simulink model "Part2_Updated_2024a"  (R2024a)
settings: Solver=FixedStepAuto  StartTime=0.0  StopTime=300  FixedStep=0.1  RelTol=1e-3
values from neighbouring files (symbols this model uses):
  Af = [0.1,0.1,0.01]    [init_Updated.m]
  Aw = [zeros(3,3), eye(3); diag(-0.3948*[1 1 1]), diag(-0.0126*[1 1 1])]    [init_Updated.m]
  B = [0,1,0,0,1,0,1,0 ... (first row only)    [init_Updated.m]
  Cw = [zeros(3) eye(3)]    [init_Updated.m]
  D = [2.6486e5, 0, 0 ... (first row only)    [init_Updated.m]
  eta0 = [0,0,0,0,0,0]'    [init_Updated.m]
  Gamma = [omega(1)^2,omega(2)^2,omega(3)^2]    [init_Updated.m]
  K1 = [diag(-3.762*[1 1 1]); diag(1.2441*[1 1 1])]    [init_Updated.m]
  K2 = diag(1.1938*[1 1 1])    [init_Updated.m]
  K3 = diag([3.57e5 3.57e5 3.57e7])    [init_Updated.m]
  K4 = 10*K3    [init_Updated.m]
  Kd = -[-885551.128894883; -1413618.40984523; -582749740.806195]    [init_Updated.m]
  Ki = -[-540.64009360768; -3153.2361136748; -1036593.12054623]    [init_Updated.m]
  Kp = -[-44440.8471205421; -174748.115243117; -56099945.0910478]    [init_Updated.m]
  M = [7.0101e6, 0, 0 ... (first row only)    [init_Updated.m]
  mu_current = 0.0001    [init_Updated.m]
  mu_current_dir = 0.001    [init_Updated.m]
  mu_dir = 0    [init_Updated.m]
  mu_speed = 0.001    [init_Updated.m]
  n = 21    [init_Updated.m]
  nu_c = 0.2    [init_Updated.m]
  omega = [2*zeta*2*pi/10,2*zeta*2*pi/10,2*zeta*2*pi/10]    [init_Updated.m]
  psi_c = n*10*pi/180    (= 3.66519142919)    [init_Updated.m]
  simulation = 2    [init_Updated.m]
  T = diag(10e3*[1 1 1])    [init_Updated.m]
  U_10 = 12    [init_Updated.m]
  U_mean = U_10 * (5 / 2 )* sqrt(kappa) * log(z / z0)    [init_Updated.m]
  Umean_angle = n*10    (= 210)    [init_Updated.m]
undefined symbols (not defined in the file or in its folder): Hoerner, thrusters, vessel, wind_coeff
libraries: simulink x11, simulink_extras x3, dspsigops x3, marine_hydro x2, marine_gnc x1
settings Model: Creator=jonbjor  LastModifiedBy=HP
settings SolverCC: AlgebraicLoopSolver=TrustRegion
settings DataIOCC: ReturnWorkspaceOutputs=off
settings DebuggingCC: UnconnectedInputMsg=warning  UnconnectedOutputMsg=warning  UnconnectedLineMsg=warning  ArithmeticOperatorsInVariantConditions=warning
settings ModelReferenceCC: EnableRefExpFcnMdlSchedulingChecks=on
settings SFSimCC: SimUseLocalCustomCode=off  CustomCodeUndefinedFunction=UseInterfaceOnly
settings RTWCC: RTWUseLocalCustomCode=off  GPUComputeCapability=3.5  DLArmComputeVersion=19.05

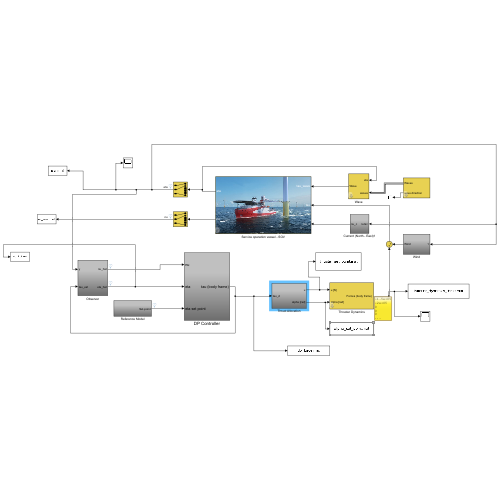
[thumbnail: Simulink's stored preview of the top-level diagram]
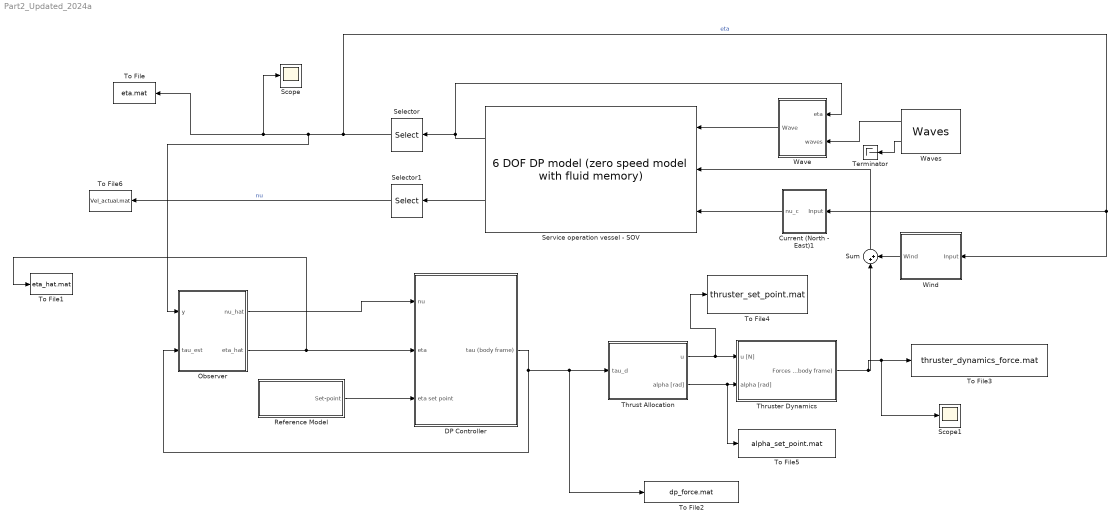
== system Part2_Updated_2024a ==
  Current (North - East)1 : Subsystem
  DP Controller : Subsystem
  Observer : Subsystem
  Reference Model : Subsystem
  Scope : Scope
  Scope1 : Scope
  Selector : Selector  InputPortWidth=6  IndexOptions=Index vector (dialog)  Indices=[1 2 6]  OutputSizes=1
  Selector1 : Selector  InputPortWidth=6  IndexOptions=Index vector (dialog)  Indices=[1 2 6]  OutputSizes=1
  Service operation vessel - SOV : marine_hydro/Hydro Library/6 DOF DP model  (zero speed model with fluid memory)  ABC=vesselABC  rho=1025  Axc=0.9*vessel.main.T*vessel.main.B  Ayc=0.9*vessel.main.T*vessel.main.Lpp  CX=1  CY_2D=Hoerner(vessel.main.B,vessel.main.T)  Bv=vessel.Bv  mask(6 DOF zero speed model){}
      mask Display:
      | image('SOV.jpg');
      | color('white'); port_label('output', 1, 'eta')
      | color('white'); port_label('output', 2, 'nu')
      | color('white'); port_label('input', 1, 'tau_wave')
      | color('white'); port_label('input', 2, 'tau')
      | color('white'); port_label('input', 3, 'nu_c')
  Sum : Sum  Inputs=|++
  Terminator : Terminator
  Thrust Allocation : Subsystem
  Thruster Dynamics : Subsystem  mask{thrusterfault=off}
      mask prompts: thrusterfault "Fault on thruster #2 and #4?"
  To File : ToFile  Filename=eta.mat  MatrixName=Track  SaveFormat=Timeseries
  To File1 : ToFile  Filename=eta_hat.mat  MatrixName=eta_hat  SaveFormat=Timeseries
  To File2 : ToFile  Filename=dp_force.mat  MatrixName=dp  SaveFormat=Timeseries
  To File3 : ToFile  Filename=thruster_dynamics_force.mat  MatrixName=thruter  SaveFormat=Timeseries
  To File4 : ToFile  Filename=thruster_set_point.mat  MatrixName=thrusterset  SaveFormat=Timeseries
  To File5 : ToFile  Filename=alpha_set_point.mat  MatrixName=alpha  SaveFormat=Timeseries
  To File6 : ToFile  Filename=Vel_actual.mat  MatrixName=Vel_actual  SaveFormat=Timeseries
  Wave : Subsystem  mask{waveforces=on}
      mask prompts: waveforces "Waveforces enabled"
  Waves : marine_gnc/Environment/Waves/Waves  spectrum_type=ITTC  disp_flag=on  plot_spectrum=off  plot_realization=off  hs=4  omega_peak=2*pi/3  psi_mean=n*10*pi/180  gamma=-1  spread=2  depth=inf  nfreq=20  ndir=10  energylim=0.005  freq_cutoff=3  dir_cutoff=0  rand_seed=123  rand_freq=on  rand_dir=on  Zeta_a=0  Omega=0  Phase=0  Wavenum=0  Psi=0
  Wind : Subsystem
  wires:
  Service operation vessel - SOV/1 -> Wave/1(eta), Selector/1
  Service operation vessel - SOV/2 -> Selector1/1
  Selector/1 -> Observer/1(y), Scope/1, To File/1, Wind/1(Input), Current (North - East)1/1(Input)  "eta"
  Thrust Allocation/1(u) -> To File4/1, Thruster Dynamics/1(u [N])
  Thrust Allocation/2(alpha [rad]) -> To File5/1, Thruster Dynamics/2(alpha [rad])
  Sum/1 -> Service operation vessel - SOV/2
  Reference Model/1(Set-point) -> DP Controller/3(eta set point)
  Waves/1 -> Wave/2(waves)
  Waves/2 -> Terminator/1
  Thruster Dynamics/1("Forces (body frame) ") -> Sum/1, Scope1/1, To File3/1
  Selector1/1 -> To File6/1  "nu"
  Observer/2(eta_hat) -> DP Controller/2(eta), To File1/1
  DP Controller/1(tau (body frame)) -> Observer/2(tau_est), To File2/1, Thrust Allocation/1(tau_d)
  Wave/1(Wave) -> Service operation vessel - SOV/1
  Current (North - East)1/1(nu_c) -> Service operation vessel - SOV/3
  Wind/1(Wind) -> Sum/2
  Observer/1(nu_hat) -> DP Controller/1(nu)

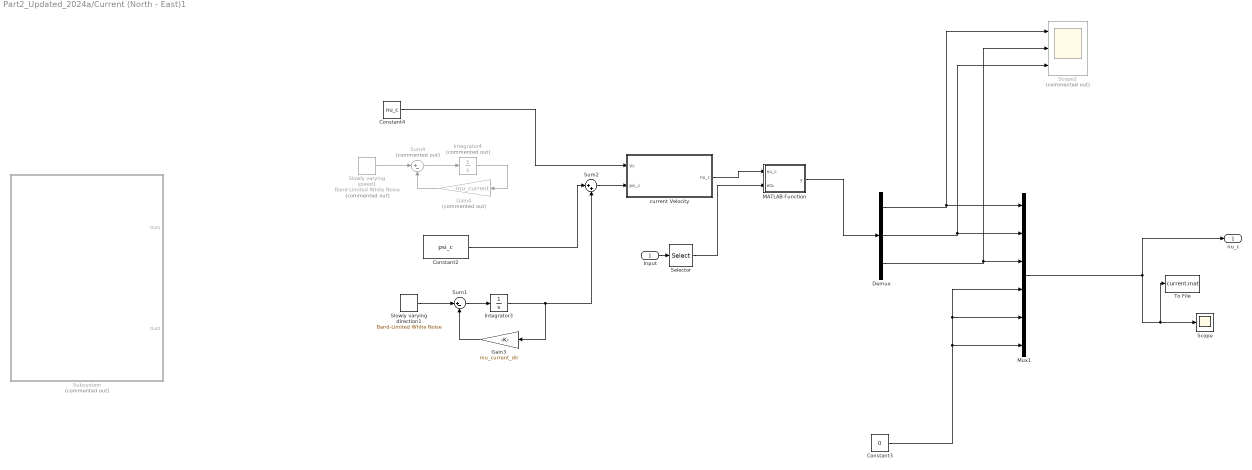
== system Part2_Updated_2024a/Current (North - East)1 ==
  Input : Inport
  Constant2 : Constant  Value=psi_c
  Constant3 : Constant  Value=0
  Constant4 : Constant  Value=nu_c
  Demux : Demux  Outputs=3
  Gain3 : Gain  Gain=mu_current_dir
  Gain4 : Gain  Commented=on  Gain=mu_current
  Integrator3 : Integrator
  Integrator4 : Integrator  Commented=on
  MATLAB Function : MATLAB Function  TreatAsAtomicUnit=on
  Mux1 : Mux  Inputs=6
  Scope : Scope
  Scope2 : Scope  Commented=on  NumInputPorts=3
  Selector : Selector  InputPortWidth=3  IndexOptions=Index vector (dialog)  Indices=[3]  OutputSizes=1
  Slowly varying speed1 : simulink/Sources/Band-Limited White Noise  Commented=on  Cov=[0.001]  Ts=0.1  seed=[23341]
  Slowly varying direction1 : simulink/Sources/Band-Limited White Noise  Cov=[0.0000001]  Ts=0.1  seed=[23341]
  Subsystem : Subsystem  Commented=on
  Sum1 : Sum  Inputs=|+-
  Sum2 : Sum  Inputs=|++
  Sum4 : Sum  Commented=on  Inputs=|+-
  To File : ToFile  Filename=current.mat  MatrixName=current  SaveFormat=Timeseries
  current Velocity : MATLAB Function  TreatAsAtomicUnit=on
  nu_c : Outport
  wires:
  Demux/1 -> Mux1/1, Scope2/1
  Demux/2 -> Mux1/2, Scope2/3
  Demux/3 -> Mux1/3, Scope2/2
  Constant3/1 -> Mux1/4, Mux1/5, Mux1/6
  current Velocity/1(nu_c) -> MATLAB Function/1(nu_c)
  Mux1/1 -> To File/1, Scope/1, nu_c/1
  MATLAB Function/1(y) -> Demux/1
  Input/1 -> Selector/1
  Sum1/1 -> Integrator3/1
  Slowly varying direction1/1 -> Sum1/1
  Integrator3/1 -> Sum2/2, Gain3/1
  Gain3/1 -> Sum1/2
  Constant2/1 -> Sum2/1
  Sum2/1 -> current Velocity/2(psi_c)
  Sum4/1 -> Integrator4/1
  Slowly varying speed1/1 -> Sum4/1
  Integrator4/1 -> Gain4/1
  Gain4/1 -> Sum4/2
  Constant4/1 -> current Velocity/1(Vc)
  Selector/1 -> MATLAB Function/2(eta)

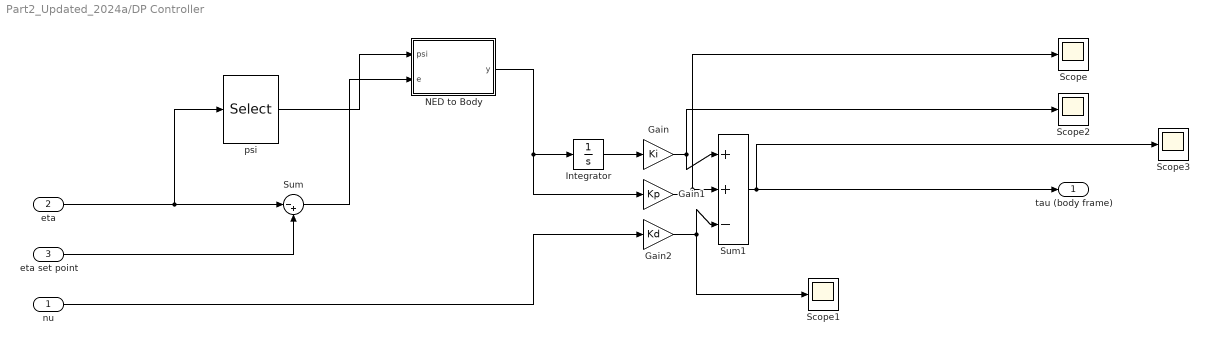
== system Part2_Updated_2024a/DP Controller ==
  nu : Inport
  eta : Inport  Port=2
  eta set point : Inport  Port=3
  Gain : Gain  Gain=Ki
  Gain1 : Gain  Gain=Kp
  Gain2 : Gain  Gain=Kd
  Integrator : Integrator
  "NED to Body " : MATLAB Function  TreatAsAtomicUnit=on
  Scope{,1..3} (4 alike) : Scope
  Sum : Sum  Inputs=|-+
  Sum1 : Sum  Inputs=|++-|
  psi : Selector  InputPortWidth=3  IndexOptions=Index vector (dialog)  Indices=[3]  OutputSizes=1
  tau (body frame) : Outport  VectorParamsAs1DForOutWhenUnconnected=off
  wires:
  Integrator/1 -> Gain/1
  eta/1 -> Sum/1, psi/1
  Sum1/1 -> tau (body frame)/1, Scope3/1
  nu/1 -> Gain2/1
  Gain/1 -> Scope2/1, Sum1/1
  Gain2/1 -> Scope1/1, Sum1/3
  Gain1/1 -> Scope/1, Sum1/2
  Sum/1 -> "NED to Body "/2(e)
  psi/1 -> "NED to Body "/1(psi)
  eta set point/1 -> Sum/2
  "NED to Body "/1(y) -> Gain1/1, Integrator/1

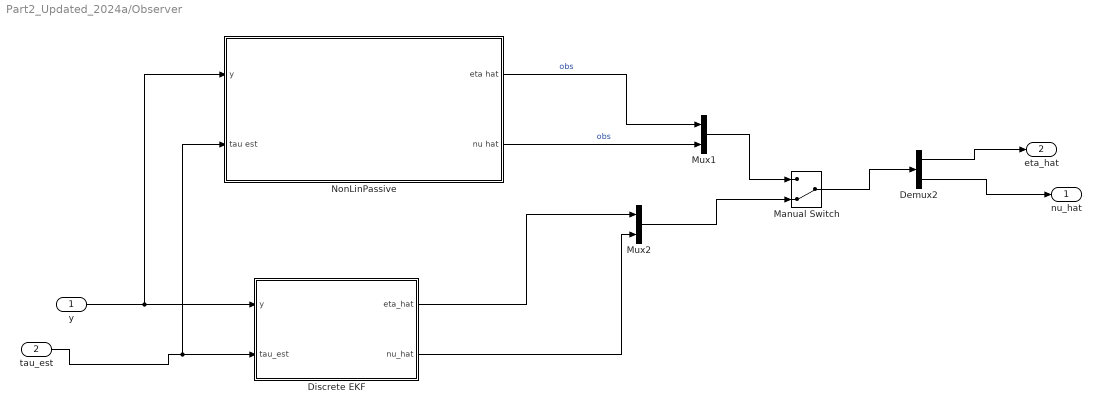
== system Part2_Updated_2024a/Observer ==
  y : Inport
  tau_est : Inport  Port=2
  Demux2 : Demux  Outputs=2
  Discrete EKF : Subsystem
  Manual Switch : ManualSwitch  CurrentSetting=0
  Mux1 : Mux  Inputs=2
  Mux2 : Mux  Inputs=2
  NonLinPassive : Subsystem
  nu_hat : Outport  VectorParamsAs1DForOutWhenUnconnected=off
  eta_hat : Outport  Port=2  VectorParamsAs1DForOutWhenUnconnected=off
  wires:
  y/1 -> Discrete EKF/1(y), NonLinPassive/1(y)
  Mux1/1 -> Manual Switch/1
  Mux2/1 -> Manual Switch/2
  Manual Switch/1 -> Demux2/1
  Demux2/1 -> eta_hat/1
  Demux2/2 -> nu_hat/1
  tau_est/1 -> Discrete EKF/2(tau_est), NonLinPassive/2(tau est)
  Discrete EKF/1(eta_hat) -> Mux2/1
  Discrete EKF/2(nu_hat) -> Mux2/2
  NonLinPassive/1(eta hat) -> Mux1/1  "obs"
  NonLinPassive/2(nu hat) -> Mux1/2  "obs"

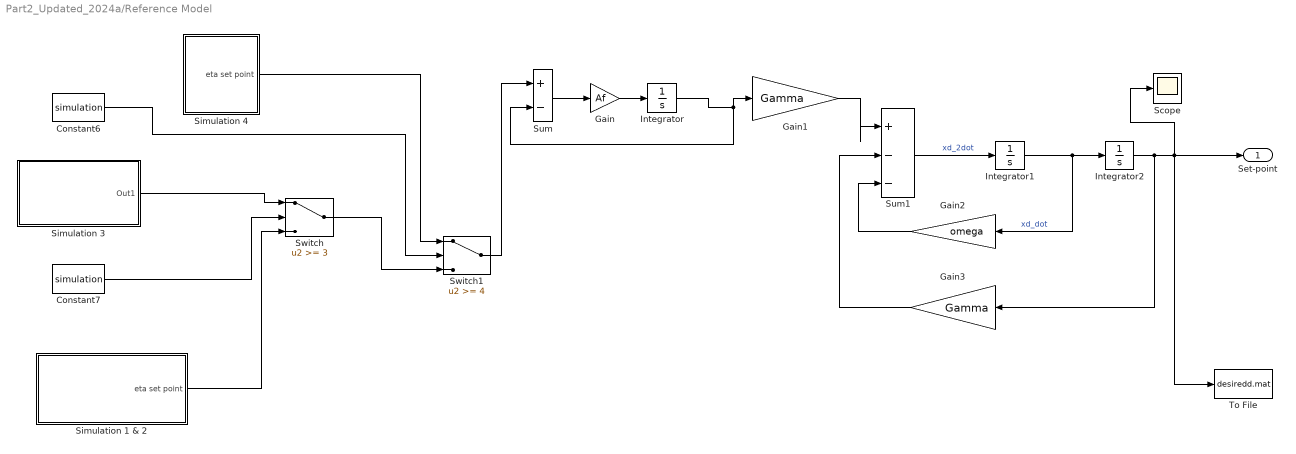
== system Part2_Updated_2024a/Reference Model ==
  Constant6 : Constant  Value=simulation
  Constant7 : Constant  Value=simulation
  Gain : Gain  Gain=Af
  Gain1 : Gain  Gain=Gamma
  Gain2 : Gain  Gain=omega
  Gain3 : Gain  Gain=Gamma
  Integrator : Integrator
  Integrator1 : Integrator
  Integrator2 : Integrator
  Scope : Scope
  Simulation 1 & 2 : Subsystem
  Simulation 3 : Subsystem
  Simulation 4 : Subsystem
  Sum : Sum  Inputs=+-
  Sum1 : Sum  Inputs=|+--
  Switch : Switch  Threshold=3  SaturateOnIntegerOverflow=off  InputSameDT=off
  Switch1 : Switch  Threshold=4  SaturateOnIntegerOverflow=off  InputSameDT=off
  To File : ToFile  Filename=desiredd.mat  MatrixName=Reff  SaveFormat=Timeseries
  Set-point : Outport  VectorParamsAs1DForOutWhenUnconnected=off
  wires:
  Gain/1 -> Integrator/1
  Sum/1 -> Gain/1
  Integrator/1 -> Sum/2, Gain1/1
  Sum1/1 -> Integrator1/1  "xd_2dot"
  Integrator1/1 -> Integrator2/1, Gain2/1  "xd_dot"
  Integrator2/1 -> Scope/1, To File/1, Set-point/1, Gain3/1
  Gain2/1 -> Sum1/3
  Gain3/1 -> Sum1/2
  Gain1/1 -> Sum1/1
  Switch1/1 -> Sum/1
  Simulation 4/1(eta set point) -> Switch1/1
  Switch/1 -> Switch1/3
  Simulation 3/1(Out1) -> Switch/1
  Constant7/1 -> Switch/2
  Constant6/1 -> Switch1/2
  Simulation 1 & 2/1(eta set point) -> Switch/3

== system Part2_Updated_2024a/Thrust Allocation ==
  tau_d : Inport
  Constant : Constant  Value=B
  MATLAB Function : MATLAB Function  TreatAsAtomicUnit=on
  unwrap : Subsystem
  u : Outport  VectorParamsAs1DForOutWhenUnconnected=off
  alpha [rad] : Outport  Port=2  VectorParamsAs1DForOutWhenUnconnected=off
  wires:
  MATLAB Function/1(u) -> u/1
  MATLAB Function/2(alpha) -> unwrap/1(In1)
  tau_d/1 -> MATLAB Function/1(tau)
  Constant/1 -> MATLAB Function/2(B)
  unwrap/1(Out1) -> alpha [rad]/1

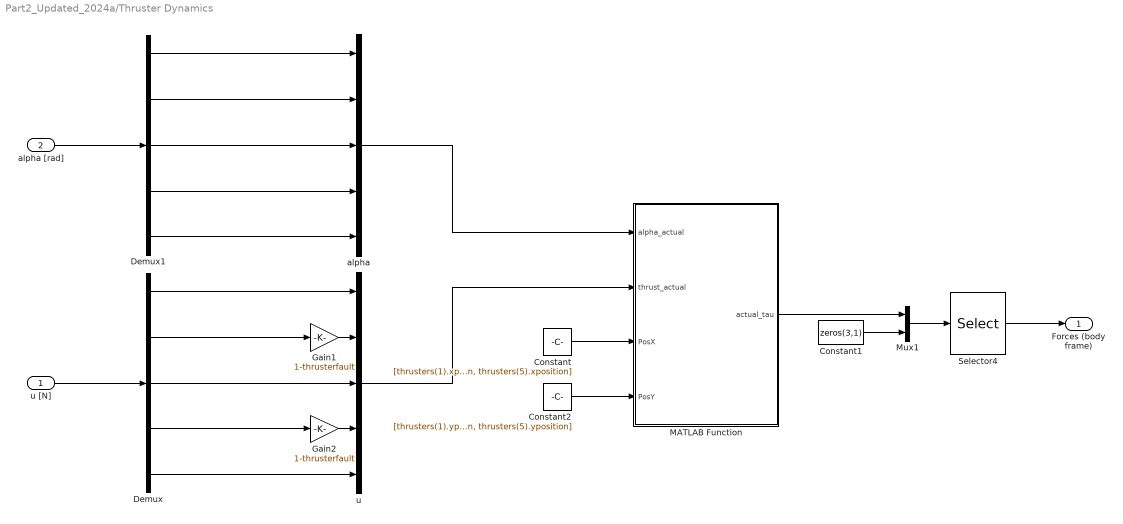
== system Part2_Updated_2024a/Thruster Dynamics ==
  u [N] : Inport
  alpha [rad] : Inport  Port=2
  Constant : Constant  Value=[thrusters(1).xposition, thrusters(2).xposition, thrusters(3).xposition, thrusters(4).xposition, thrusters(5).xposition]
  Constant1 : Constant  Value=zeros(3,1)
  Constant2 : Constant  Value=[thrusters(1).yposition, thrusters(2).yposition, thrusters(3).yposition, thrusters(4).yposition, thrusters(5).yposition]
  Demux : Demux  Outputs=5
  Demux1 : Demux  Outputs=5
  Gain1 : Gain  Gain=1-thrusterfault
  Gain2 : Gain  Gain=1-thrusterfault
  MATLAB Function : MATLAB Function  TreatAsAtomicUnit=on
  Mux1 : Mux  Inputs=2
  Selector4 : Selector  InputPortWidth=6  IndexOptions=Index vector (dialog)  Indices=[1 2 4 5 6 3]  OutputSizes=1
  alpha : Mux  Inputs=5
  u : Mux  Inputs=5
  "Forces (body frame) " : Outport  VectorParamsAs1DForOutWhenUnconnected=off
  wires:
  Mux1/1 -> Selector4/1
  Constant1/1 -> Mux1/2
  Selector4/1 -> "Forces (body frame) "/1
  Gain1/1 -> u/2
  u [N]/1 -> Demux/1
  alpha [rad]/1 -> Demux1/1
  Constant/1 -> MATLAB Function/3(PosX)
  Constant2/1 -> MATLAB Function/4(PosY)
  u/1 -> MATLAB Function/2(thrust_actual)
  alpha/1 -> MATLAB Function/1(alpha_actual)
  MATLAB Function/1(actual_tau) -> Mux1/1
  Demux1/1 -> alpha/1
  Gain2/1 -> u/4
  Demux/1 -> u/1
  Demux/2 -> Gain1/1
  Demux/3 -> u/3
  Demux/4 -> Gain2/1
  Demux/5 -> u/5
  Demux1/2 -> alpha/2
  Demux1/4 -> alpha/4
  Demux1/5 -> alpha/5
  Demux1/3 -> alpha/3

== system Part2_Updated_2024a/Wave ==
  eta : Inport
  waves : Inport  Port=2
  Gain : Gain  Gain=waveforces
  Sum : Sum
  Wave loads (U=0) : marine_hydro/Hydro Library/Wave loads (U=0)  SystemSampleTime=-1  VariantActivationTime=update diagram  AllowFlexibleInterface=on  Latency=0  AutoFrameSizeCalculation=off
      settings: SourceProductName=MSS Hydro
  Wave : Outport  VectorParamsAs1DForOutWhenUnconnected=off
  wires:
  eta/1 -> Wave loads (U=0)/1
  waves/1 -> Wave loads (U=0)/2
  Sum/1 -> Gain/1
  Wave loads (U=0)/1 -> Sum/1
  Wave loads (U=0)/2 -> Sum/2
  Gain/1 -> Wave/1

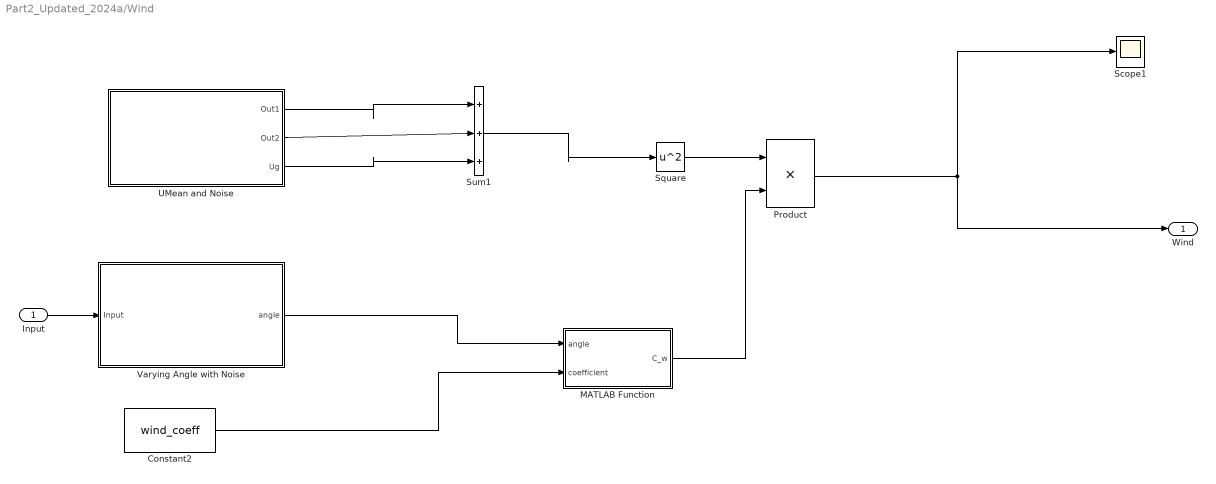
== system Part2_Updated_2024a/Wind ==
  Input : Inport
  Constant2 : Constant  Value=wind_coeff
  MATLAB Function : MATLAB Function  TreatAsAtomicUnit=on
  Product : Product
  Scope1 : Scope
  Square : Math  Operator=square
  Sum1 : Sum  Inputs=|+++
  UMean and Noise : Subsystem
  Varying Angle with Noise : Subsystem
  Wind : Outport  VectorParamsAs1DForOutWhenUnconnected=off
  wires:
  Sum1/1 -> Square/1
  Square/1 -> Product/1
  Constant2/1 -> MATLAB Function/2(coefficient)
  MATLAB Function/1(C_w) -> Product/2
  UMean and Noise/1(Out1) -> Sum1/1
  UMean and Noise/2(Out2) -> Sum1/2
  Product/1 -> Wind/1, Scope1/1
  Varying Angle with Noise/1(angle) -> MATLAB Function/1(angle)
  UMean and Noise/3(Ug) -> Sum1/3
  Input/1 -> Varying Angle with Noise/1(Input)

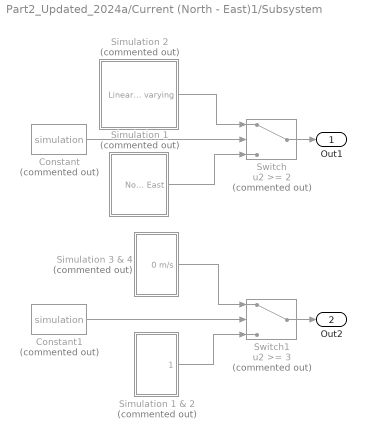
== system Part2_Updated_2024a/Current (North - East)1/Subsystem ==
  Constant : Constant  Commented=on  Value=simulation
  Constant1 : Constant  Commented=on  Value=simulation
  Simulation 1 : Subsystem  Commented=on
  Simulation 1 & 2 : Subsystem  Commented=on
  Simulation 2 : Subsystem  Commented=on
  Simulation 3 & 4 : Subsystem  Commented=on
  Switch : Switch  Commented=on  Threshold=2  SaturateOnIntegerOverflow=off  InputSameDT=off
  Switch1 : Switch  Commented=on  Threshold=3  SaturateOnIntegerOverflow=off  InputSameDT=off
  Out1 : Outport
  Out2 : Outport  Port=2
  wires:
  Simulation 3 & 4/1(0 m/s) -> Switch1/1
  Constant1/1 -> Switch1/2
  Switch1/1 -> Out2/1
  Constant/1 -> Switch/2
  Simulation 1 & 2/1(0.5 m/s) -> Switch1/3
  Simulation 1/1(North East) -> Switch/3
  Simulation 2/1(Linearly varying) -> Switch/1
  Switch/1 -> Out1/1

== system Part2_Updated_2024a/Observer/Discrete EKF ==
  y : Inport
  tau_est : Inport  Port=2
  MATLAB Function : MATLAB Function  TreatAsAtomicUnit=on
  Memory : Memory  InitialCondition=zeros(15,15)
  Memory1 : Memory  InitialCondition=zeros(15,1)
  eta_hat : Outport
  nu_hat : Outport  Port=2
  wires:
  y/1 -> MATLAB Function/1(y)
  tau_est/1 -> MATLAB Function/2(tau_est)
  MATLAB Function/1(eta_est) -> eta_hat/1
  MATLAB Function/2(nu_est) -> nu_hat/1
  MATLAB Function/3(x_bar) -> Memory1/1
  MATLAB Function/4(P_bar) -> Memory/1
  Memory/1 -> MATLAB Function/4("P_bar ")
  Memory1/1 -> MATLAB Function/3("x_bar ")

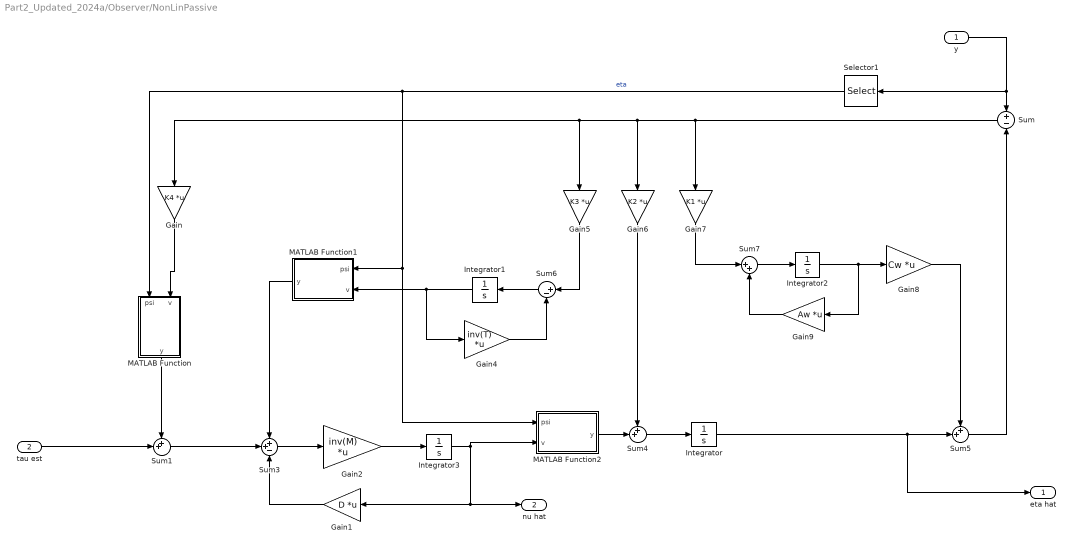
== system Part2_Updated_2024a/Observer/NonLinPassive ==
  y : Inport
  tau est : Inport  Port=2
  Gain : Gain  Gain=K4  Multiplication=Matrix(K*u)
  Gain1 : Gain  Gain=D  Multiplication=Matrix(K*u)
  Gain2 : Gain  Gain=inv(M)  Multiplication=Matrix(K*u)
  Gain4 : Gain  Gain=inv(T)  Multiplication=Matrix(K*u)
  Gain5 : Gain  Gain=K3  Multiplication=Matrix(K*u)
  Gain6 : Gain  Gain=K2  Multiplication=Matrix(K*u)
  Gain7 : Gain  Gain=K1  Multiplication=Matrix(K*u)
  Gain8 : Gain  Gain=Cw  Multiplication=Matrix(K*u)
  Gain9 : Gain  Gain=Aw  Multiplication=Matrix(K*u)
  Integrator{,1..3} (4 alike) : Integrator
  MATLAB Function : MATLAB Function  TreatAsAtomicUnit=on
  MATLAB Function1 : MATLAB Function  TreatAsAtomicUnit=on
  MATLAB Function2 : MATLAB Function  TreatAsAtomicUnit=on
  Selector1 : Selector  InputPortWidth=3  IndexOptions=Index vector (dialog)  Indices=3  OutputSizes=1
  Sum : Sum  Inputs=+|-
  Sum1 : Sum  Inputs=++|
  Sum3 : Sum  Inputs=++-
  Sum4 : Sum  Inputs=++|
  Sum5 : Sum  Inputs=++|
  Sum6 : Sum  Inputs=|+-
  Sum7 : Sum  Inputs=|++
  eta hat : Outport
  nu hat : Outport  Port=2
  wires:
  Sum4/1 -> Integrator/1
  Sum6/1 -> Integrator1/1
  Gain4/1 -> Sum6/2
  Gain2/1 -> Integrator3/1
  Sum5/1 -> Sum/2
  Sum7/1 -> Integrator2/1
  Integrator3/1 -> MATLAB Function2/2(v), nu hat/1, Gain1/1
  Gain/1 -> MATLAB Function/2(v)
  Sum3/1 -> Gain2/1
  Sum/1 -> Gain7/1, Gain6/1, Gain5/1, Gain/1
  Gain6/1 -> Sum4/1
  y/1 -> Selector1/1, Sum/1
  Gain8/1 -> Sum5/1
  Integrator1/1 -> MATLAB Function1/2(v), Gain4/1
  Gain5/1 -> Sum6/1
  tau est/1 -> Sum1/2
  Gain9/1 -> Sum7/2
  Integrator2/1 -> Gain9/1, Gain8/1
  Gain1/1 -> Sum3/3
  Gain7/1 -> Sum7/1
  Selector1/1 -> MATLAB Function/1(psi), MATLAB Function2/1(psi), MATLAB Function1/1(psi)  "eta"
  MATLAB Function1/1(y) -> Sum3/1
  Integrator/1 -> eta hat/1, Sum5/2
  Sum1/1 -> Sum3/2
  MATLAB Function2/1(y) -> Sum4/2
  MATLAB Function/1(y) -> Sum1/1

== system Part2_Updated_2024a/Reference Model/Simulation 1 & 2 ==
  6 to 3 DOF : Selector  InputPortWidth=6  IndexOptions=Index vector (dialog)  Indices=[1 2 6]  OutputSizes=1
  Set-point : Constant  Value=eta0
  eta set point : Outport
  wires:
  Set-point/1 -> 6 to 3 DOF/1
  6 to 3 DOF/1 -> eta set point/1

== system Part2_Updated_2024a/Reference Model/Simulation 3 ==
  East : Step  After=10  SampleTime=0
  Heading : Step  After=3*pi/2  SampleTime=0
  Mux : Mux  Inputs=3
  North : Step  After=10  SampleTime=0
  Out1 : Outport
  wires:
  North/1 -> Mux/1
  East/1 -> Mux/2
  Mux/1 -> Out1/1
  Heading/1 -> Mux/3

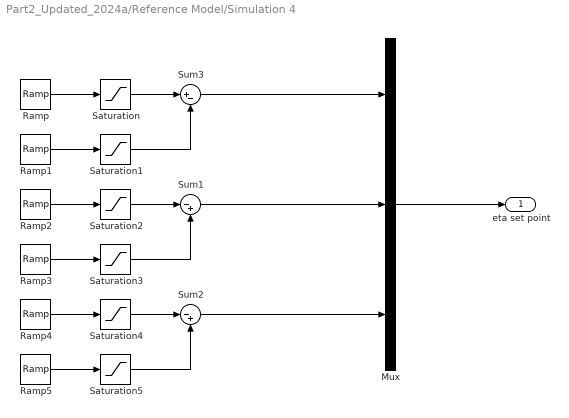
== system Part2_Updated_2024a/Reference Model/Simulation 4 ==
  Mux : Mux  Inputs=3
  Ramp : simulink/Sources/Ramp  slope=0.5  start=10  InitialOutput=0
  Ramp1 : simulink/Sources/Ramp  slope=0.5  start=1200  InitialOutput=0
  Ramp2 : simulink/Sources/Ramp  slope=0.5  start=10  InitialOutput=0
  Ramp3 : simulink/Sources/Ramp  slope=0.5  start=1200  InitialOutput=0
  Ramp4 : simulink/Sources/Ramp  slope=0.9  start=600  InitialOutput=0
  Ramp5 : simulink/Sources/Ramp  slope=0.9  start=1200  InitialOutput=0
  Saturation{,1..3} (4 alike) : Saturate  UpperLimit=50  LowerLimit=0
  Saturation4 : Saturate  UpperLimit=pi/4  LowerLimit=0
  Saturation5 : Saturate  UpperLimit=pi/4  LowerLimit=0
  Sum1 : Sum  Inputs=|-+
  Sum2 : Sum  Inputs=|-+
  Sum3 : Sum  Inputs=|+-
  eta set point : Outport
  wires:
  Ramp4/1 -> Saturation4/1
  Ramp5/1 -> Saturation5/1
  Saturation3/1 -> Sum1/2
  Saturation5/1 -> Sum2/2
  Saturation4/1 -> Sum2/1
  Ramp2/1 -> Saturation2/1
  Saturation2/1 -> Sum1/1
  Ramp3/1 -> Saturation3/1
  Saturation1/1 -> Sum3/2
  Sum3/1 -> Mux/1
  Saturation/1 -> Sum3/1
  Sum1/1 -> Mux/2
  Ramp1/1 -> Saturation1/1
  Ramp/1 -> Saturation/1
  Sum2/1 -> Mux/3
  Mux/1 -> eta set point/1

== system Part2_Updated_2024a/Thrust Allocation/unwrap ==
  In1 : Inport
  Demux : Demux  Outputs=5
  Mux : Mux  Inputs=5
  Unwrap : dspsigops/Unwrap  tol=pi  InputProcessing=Columns as channels (frame based)  running=off
  Unwrap1 : dspsigops/Unwrap  tol=pi  InputProcessing=Columns as channels (frame based)  running=off
  Unwrap2 : dspsigops/Unwrap  tol=pi  InputProcessing=Columns as channels (frame based)  running=off
  Out1 : Outport
  wires:
  Unwrap/1 -> Mux/5
  Demux/5 -> Unwrap/1
  Demux/3 -> Unwrap2/1
  Demux/2 -> Mux/2
  Demux/1 -> Mux/1
  Demux/4 -> Unwrap1/1
  Unwrap1/1 -> Mux/4
  Unwrap2/1 -> Mux/3
  Mux/1 -> Out1/1
  In1/1 -> Demux/1

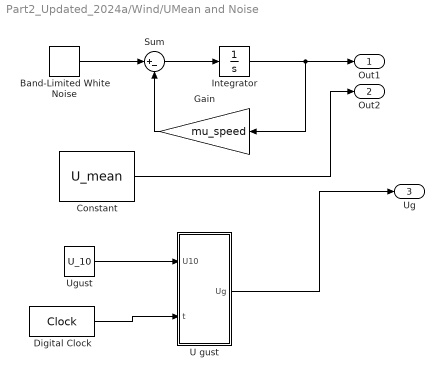
== system Part2_Updated_2024a/Wind/UMean and Noise ==
  Band-Limited White Noise : simulink/Sources/Band-Limited White Noise  Cov=U_w  Ts=0.1  seed=[23341]
  Constant : Constant  Value=U_mean
  Digital Clock : DigitalClock
  Gain : Gain  Gain=mu_speed
  Integrator : Integrator
  Sum : Sum  Inputs=|+-
  U gust : MATLAB Function  TreatAsAtomicUnit=on
  Ugust : Constant  Value=U_10
  Out1 : Outport
  Out2 : Outport  Port=2
  Ug : Outport  Port=3
  wires:
  Integrator/1 -> Out1/1, Gain/1
  Gain/1 -> Sum/2
  Band-Limited White Noise/1 -> Sum/1
  Sum/1 -> Integrator/1
  Constant/1 -> Out2/1
  Digital Clock/1 -> U gust/2(t)
  Ugust/1 -> U gust/1(U10)
  U gust/1(Ug) -> Ug/1

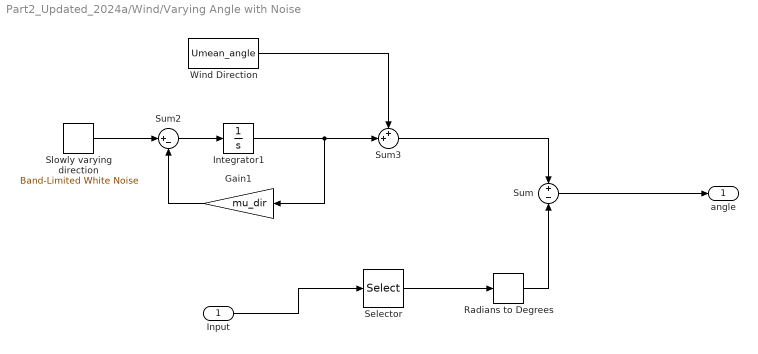
== system Part2_Updated_2024a/Wind/Varying Angle with Noise ==
  Input : Inport
  Gain1 : Gain  Gain=mu_dir
  Integrator1 : Integrator
  Radians to Degrees : simulink_extras/Transformations/Radians to Degrees
  Selector : Selector  InputPortWidth=3  IndexOptions=Index vector (dialog)  Indices=3  OutputSizes=1
  Slowly varying direction : simulink/Sources/Band-Limited White Noise  Cov=[0.0000001]  Ts=0.1  seed=[23341]
  Sum : Sum  Inputs=+-
  Sum2 : Sum  Inputs=|+-
  Sum3 : Sum  Inputs=++|
  Wind Direction : Constant  Value=Umean_angle
  angle : Outport
  wires:
  Sum2/1 -> Integrator1/1
  Integrator1/1 -> Sum3/2, Gain1/1
  Slowly varying direction/1 -> Sum2/1
  Gain1/1 -> Sum2/2
  Input/1 -> Selector/1
  Wind Direction/1 -> Sum3/1
  Sum3/1 -> Sum/1
  Selector/1 -> Radians to Degrees/1
  Sum/1 -> angle/1
  Radians to Degrees/1 -> Sum/2

== system Part2_Updated_2024a/Current (North - East)1/Subsystem/Simulation 1 ==
  Degrees to Radians : simulink_extras/Transformations/Degrees to Radians
  Psi_c (deg) : Constant  Value=135  VectorParams1D=off  SampleTime=-1
  North East : Outport
  wires:
  Degrees to Radians/1 -> North East/1
  Psi_c (deg)/1 -> Degrees to Radians/1

== system Part2_Updated_2024a/Current (North - East)1/Subsystem/Simulation 1 & 2 ==
  Nu_c (m/s) : Constant  Value=nu_c  VectorParams1D=off  SampleTime=-1
  0.5 m/s : Outport
  wires:
  Nu_c (m/s)/1 -> 0.5 m/s/1

== system Part2_Updated_2024a/Current (North - East)1/Subsystem/Simulation 2 ==
  Degrees to Radians1 : simulink_extras/Transformations/Degrees to Radians
  Ramp : simulink/Sources/Ramp  slope=0.3  start=0  InitialOutput=180
  Saturation : Saturate  UpperLimit=270  LowerLimit=180
  Scope : Scope
  Linearly varying : Outport
  wires:
  Degrees to Radians1/1 -> Scope/1, Linearly varying/1
  Saturation/1 -> Degrees to Radians1/1
  Ramp/1 -> Saturation/1

== system Part2_Updated_2024a/Current (North - East)1/Subsystem/Simulation 3 & 4 ==
  Constant2 : Constant  Value=0
  0 m/s : Outport
  wires:
  Constant2/1 -> 0 m/s/1

== matlab function Part2_Updated_2024a/Observer/Discrete EKF/MATLAB Function ==
  data: y input; eta_est output; tau_est input; nu_est output; x_bar input; P_bar input; x_bar output; P_bar output
function [eta_est,nu_est,x_bar,P_bar] = EKF(y,tau_est,x_bar,P_bar)

T_pi = 7; 
omega_i = (2*pi)/T_pi; % Wave peak frequency
T = diag([1, 1, 1])*1000; % Diagonal matrix of bias time constant (3x3)
T_inv = inv(T); % (3x3)
M = [7.0101e6 0 0;0 8.5190e6 4.7187e5;0 4.7187e5 3.7973e9]; % Inertia matrix (3x3)
M_inv = inv(M); % (3x3)
zeta = 0.1; % zeta = 0.05 - 0.1
A_w = [diag([0, 0, 0]),diag([1, 1, 1]);-omega_i^2*diag([1, 1, 1]),-2*zeta*omega_i*diag([1, 1, 1])]; % Wave parameters (6x6), depend on omega_i
C_w = [diag([0, 0, 0]),diag([1, 1, 1])]; % Constant matrix (6x3)
D = [2.6486e5 0 0;0 8.8164e5 0;0 0 3.3774e8]; % Linear damping matrix (3x3)

B = [zeros(6,3);zeros(3,3);zeros(3,3);M_inv]; % (15x3)
H = [C_w,eye(3),zeros(3,3),zeros(3,3)]; % (3x15)
E_w = [zeros(3,3);eye(3)]; % (3x6)
E_b = eye(3); % (3x3)
E = [E_w zeros(6,3);zeros(3,3) zeros(3,3);zeros(3,3) E_b;zeros(3,3) zeros(3,3)]; % (15x6)
u = [tau_est(1);tau_est(2);tau_est(3)]; % (3x1)

R = diag([0.00001,0.00001,0.01*pi/180])*10e-4; %tune later %measurement

Q = diag([0.1,0.1,pi/180,1e6,1e6,1e9])*10e3;

h = 0.1; % REMEMBER TO PUT THIS AS THE SAME AS IN THE SIMULATIONS!
psi = y(3);

K = P_bar * H' * inv(H * P_bar * H' + R); % Kalman gain matrix (15x3)
x_hat = x_bar + K * (y - H * x_bar); % State estimation corrector (15x1)

epsilon_est = [x_hat(1);x_hat(2);x_hat(3);x_hat(4);x_hat(5);x_hat(6)]; % (6x1)
eta_est = [x_hat(7);x_hat(8);x_hat(9)]; % (3x1)
b_est = [x_hat(10);x_hat(11);x_hat(12)]; % (3x1)
nu_est = [x_hat(13);x_hat(14);x_hat(15)]; %(3x1)

P_hat = (eye(15) - K * H) * P_bar * (eye(15) - K * H)' + K * R * K'; % Error covariance corrector (15x15)

% Setting up the Jacobian
J11 = A_w; % Derivative of f1(x,u) with respect to epsilon
J12 = zeros(6,3); % Derivative of f1(x,u) with respect to eta
J13 = zeros(6,3); % Derivative of f1(x,u) with respect to b
J14 = zeros(6,3); % Derivative of f1(x,u) with respect to nu
J21 = zeros(3,6); % Derivative of f2(x,u) with respect to epsilon
J22 = [zeros(3,2),[-nu_est(1)*sin(psi)-nu_est(2)*cos(psi);nu_est(1)*cos(psi)-nu_est(2)*sin(psi);0]]; % Derivative of f2(x,u) with respect to eta
J23 = zeros(3,3); % Derivative of f2(x,u) with respect to b
J24 = [cos(psi) -sin(psi) 0;sin(psi) cos(psi) 0;0 0 1]; % Derivative of f2(x,u) with respect to nu
J31 = zeros(3,6); % Derivative of f3(x,u) with respect to epsilon
J32 = zeros(3,3); % Derivative of f3(x,u) with respect to eta
J33 = T_inv; % Derivative of f3(x,u) with respect to b
J34 = zeros(3,3); % Derivative of f3(x,u) with respect to nu
J41 = zeros(3,6); % Derivative of f4(x,u) with respect to epsilon
J42 = [zeros(3,2),M_inv*[-sin(psi) cos(psi) 0;-cos(psi) -sin(psi) 0;0 0 0]*b_est]; % Derivative of f4(x,u) with respect to eta
J43 = M_inv*[cos(psi) sin(psi) 0;-sin(psi) cos(psi) 0;0 0 1]; % Derivative of f4(x,u) with respect to b
J44 = -M_inv*D; % Derivative of f4(x,u) with respect to nu

Jacobian = [J11 J12 J13 J14;J21 J22 J23 J24;J31 J32 J33 J34;J41 J42 J43 J44];

Phi = eye(15) + h * Jacobian;
Gamma = h * E;

F_xhat_u = [A_w*epsilon_est;[cos(psi) -sin(psi) 0;sin(psi) cos(psi) 0;0 0 1]*nu_est;-T_inv*b_est;M_inv*(-D*nu_est + [cos(psi) -sin(psi) 0;sin(psi) cos(psi) 0;0 0 1]'*b_est)];

x_bar = x_hat + h * (F_xhat_u +  B * u); % State estimation predictor (15x1)
P_bar = Phi * P_hat * Phi' + Gamma * Q * Gamma'; % Error covariance predictor (15x15)

end

== matlab function Part2_Updated_2024a/Wind/MATLAB Function ==
  data: angle input; C_w output; coefficient input
function C_w = fcn(angle, coefficient)

angle = mod(angle,360);
i = round(angle/10)+1;

C_w = [coefficient(i,2);
    coefficient(i,3);
    coefficient(i,4);
    coefficient(i,5);
    coefficient(i,6);
    coefficient(i,7)];

== matlab function Part2_Updated_2024a/Current (North - East)1/MATLAB Function ==
  data: nu_c input; y output; eta input
function y = fcn(nu_c,eta)
R=[cos(eta), -sin(eta) , 0;
  sin(eta), cos(eta),  0;
  0 ,0 , 1];


nu_c=R'*nu_c

y = nu_c;

== matlab function Part2_Updated_2024a/Wind/UMean and Noise/U gust ==
  data: U10 input; Ug output; t input
function Ug = fcn(U10, t)
    f = linspace(10e-4, 1, 500);
    delta = f(2)-f(1);
    Ug = 0;
    L = 1800;
    kappa = 0.0026;
    for i = length(f)
        f_tilde = L*f(i)/U10;
        S = (4*kappa*L*U10)/((2+f_tilde^2)^(5/6));
        epsilon = rand(1)*2*pi;
        Ug = Ug + sqrt(2*S*delta)*cos(2*pi*f(i)*t+epsilon);
    end
end

== matlab function Part2_Updated_2024a/Thruster Dynamics/MATLAB Function ==
  data: alpha_actual input; thrust_actual input; actual_tau output; PosX input; PosY input
function actual_tau   = fcn(alpha_actual,thrust_actual,PosX,PosY)

    Alpha_surge =[cos(alpha_actual(1)) cos(alpha_actual(2)) cos(alpha_actual(3)) cos(alpha_actual(4)) cos(alpha_actual(5))];  
    Alpha_sway = [sin(alpha_actual(1)) sin(alpha_actual(2)) sin(alpha_actual(3)) sin(alpha_actual(4)) sin(alpha_actual(5))];
    Alpha_yaw = [sin(alpha_actual(1))*PosX(1)-cos(alpha_actual(1))*PosY(1) sin(alpha_actual(2))*PosX(2)-cos(alpha_actual(2))*PosY(2) ...
                 sin(alpha_actual(3))*PosX(3)-cos(alpha_actual(3))*PosY(3) sin(alpha_actual(4))*PosX(4)-cos(alpha_actual(4))*PosY(4) ...
                 sin(alpha_actual(5))*PosX(5)-cos(alpha_actual(5))*PosY(5)];

    actual_tau = [Alpha_surge; Alpha_sway; Alpha_yaw]*thrust_actual;
end

== matlab function Part2_Updated_2024a/Current (North - East)1/current Velocity ==
  data: Vc input; nu_c output; psi_c input
function nu_c = compute_nu_c(Vc, psi_c)
    % psi_c - heading angle in radians
    nu_c = [Vc * cos(psi_c); Vc * sin(psi_c); 0];
end

== matlab function Part2_Updated_2024a/DP Controller/NED to Body  ==
  data: psi input; e input; y output
function y = fcn(psi,e)
R_b_n= [cos(psi), sin(psi), 0;
            -sin(psi), cos(psi),0;
             0, 0,1];


y = R_b_n*e;

== matlab function Part2_Updated_2024a/Thrust Allocation/MATLAB Function ==
  settings: updateMethod=DISCRETE
  data: tau input; u output; alpha output; B input
% function [u, alpha] = fcn(tau, B)
% 
% Td0 = zeros(8,1);
% 
% persistent u_l
% 
% if isempty(u_l)
%     u_l = Td0;
% end
% 
% h = 0.1;
% 
% 
% u_max = 1000 * [125, 150, 150, 125, 300, 300, 300, 300]';
% u_min = -u_max;
% 
% time_to_max = [8,8,8,8,10,10,10,10]';
% delta_max = u_max./time_to_max*h;
% delta_min = -delta_max;
% rpm_max= [NaN,2,2,NaN,2,2,2,2]';
% rpm_min= -rpm_max;
% 
% 
% lim_max = delta_max + u_l;
% lim_min = delta_min + u_l;
% 
% sWeight = 1e5;
% H =  2*diag([2,2,2,2,0.9,0.9,0.9,0.9,sWeight,sWeight,sWeight*10]);
% 
% A_eq = [B, -eye(3)];
% 
% A = [-eye(8) ,  zeros(8,3);
%       eye(8) ,   zeros(8,3)];
% 
% b_eq = tau;
% b = [-(max(u_min, lim_min)); 
%     min(u_max,lim_max)];
% 
% f = zeros(length(H),1);
% x = ones(11,1);
% x0 = ones(11,1);
% coder.extrinsic('quadprog');
% coder.extrinsic('optimoptions');
% options = optimoptions('quadprog',...
%  'Algorithm','active-set','Display','off','Steptolerance',...
% 1e-30,'OptimalityTolerance',1e+3);
% x = quadprog(H,f,A,b,A_eq,b_eq, [],[],x0,options);
% Td = x(1:8);
% 
% 
% 
% u4x = Td(6);
% u5x = Td(8);
% 
% u1 = Td(1);
% %u2=0;
% u2 = sqrt(Td(3)^2+Td(2)^2);
% u3 = Td(4);
% %u4=0;
% u4 = sqrt(Td(5)^2 + Td(6)^2);
% u5 = sqrt(Td(7)^2 + Td(8)^2);
% 
% a1 = pi/2;
% % a2=0;
% a2 = atan2(Td(3),Td(2));
% a3 = pi/2; 
% % a4=0;
% a4 = atan2(Td(6), Td(5));
% a5 = atan2(Td(8), Td(7));
% u_l = Td(1:8);
% 
% alpha = [a1 a2 a3 a4 a5]';
% u = [u1 u2 u3 u4 u5]';
% 
function [u, alpha] = fcn(tau, B)
    Td0 = zeros(8,1);
    persistent u_l

    if isempty(u_l)
        u_l = Td0;
    end

    h = 0.1;  % Time step

    % Define max and min thrust force values
    u_max = 1000 * [125, 150, 150, 125, 300, 300, 300, 300]';
    u_min = -u_max;

    % Define max and min thrust rate of change (to control rapid changes)
    time_to_max = [8,8,8,8,10,10,10,10]';
    delta_max = u_max ./ time_to_max * h;
    delta_min = -delta_max;

    % Define RPM constraints (in terms of corresponding force limits)
    rpm_max = [NaN, 2, 2, NaN, 2, 2, 2, 2]';
    rpm_min = -rpm_max;

    % Apply thrust rate limits
    lim_max = delta_max + u_l;
    lim_min = delta_min + u_l;

    % Weighting for slack variables (for feasibility in optimization)
    sWeight = 1e5;
    H = 2 * diag([2, 2, 2, 2, 0.9, 0.9, 0.9, 0.9, sWeight, sWeight, sWeight * 10]);

    % Equality constraint for force balance
    A_eq = [B, -eye(3)];
    b_eq = tau;

    % Inequality constraints for thrust limits
    A = [-eye(8), zeros(8,3); 
          eye(8), zeros(8,3)];

    % Adjust thrust limits based on RPM constraints
    for i = 1:length(rpm_max)
        if ~isnan(rpm_max(i))
            % Adjust the max thrust force based on the max RPM
            u_max(i) = min(u_max(i), rpm_max(i) * h);
            u_min(i) = max(u_min(i), rpm_min(i) * h);
        end
    end

    % Update inequality bounds
    b = [-(max(u_min, lim_min)); 
          min(u_max, lim_max)];

    % Optimization parameters
    f = zeros(length(H), 1);
    x0 = ones(11, 1);
    
    % Define options for the optimizer
    options = optimoptions('quadprog', 'Algorithm', 'active-set', ...
        'Display', 'off', 'StepTolerance', 1e-30, 'OptimalityTolerance', 1e+3);
    
    % Solve using quadprog
    x = quadprog(H, f, A, b, A_eq, b_eq, [], [], x0, options);
    
    % Extract thrust forces and convert them to desired format
    Td = x(1:8);
    
    % Calculate forces and RPMs for each thruster
    u1 = Td(1);
    u2 = sqrt(Td(3)^2 + Td(2)^2);
    u3 = Td(4);
    u4 = sqrt(Td(5)^2 + Td(6)^2);
    u5 = sqrt(Td(7)^2 + Td(8)^2);

    % Calculate azimuth angles for each thruster
    a1 = pi / 2;
    a2 = atan2(Td(3), Td(2));
    a3 = pi / 2; 
    a4 = atan2(Td(6), Td(5));
    a5 = atan2(Td(8), Td(7));

    % Update persistent state for next time step
    u_l = Td(1:8);

    % Return results
    alpha = [a1 a2 a3 a4 a5]';
    u = [u1 u2 u3 u4 u5]';
end

== matlab function Part2_Updated_2024a/Observer/NonLinPassive/MATLAB Function ==
  data: psi input; v input; y output
function y = fcn(psi,v)
R=[cos(psi), -sin(psi) , 0;
  sin(psi), cos(psi),  0;
  0 ,0 , 1];

y = R*v;

== matlab function Part2_Updated_2024a/Observer/NonLinPassive/MATLAB Function1 ==
  data: psi input; v input; y output
function y = fcn(psi,v)
R=[cos(psi), -sin(psi) , 0;
  sin(psi), cos(psi),  0;
  0 ,0 , 1];

y = R*v;

== matlab function Part2_Updated_2024a/Observer/NonLinPassive/MATLAB Function2 ==
  data: psi input; v input; y output
function y = fcn(psi,v)
R=[cos(psi), -sin(psi) , 0;
  sin(psi), cos(psi),  0;
  0 ,0 , 1];


y = R*v;
